simulink model "evitar_choque2023v"  (R2023b)
settings: Solver=VariableStepAuto  StartTime=0.0  StopTime=10.0  RelTol=1e-3
settings Model: Creator=Usuario_UMA  LastModifiedBy=juana

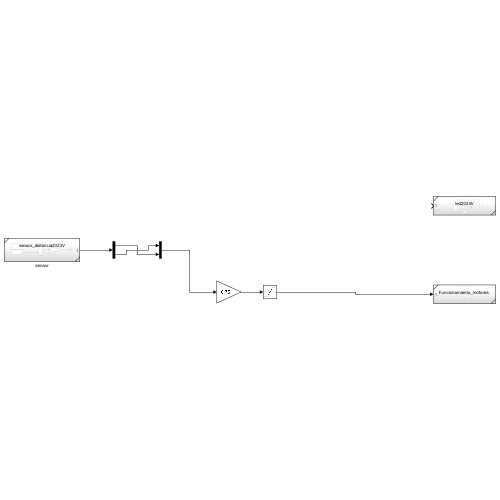
[thumbnail: Simulink's stored preview of the top-level diagram]
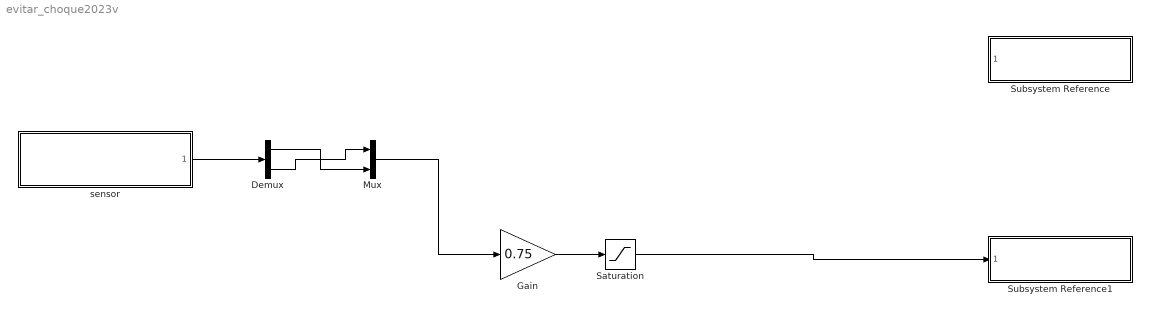
== system evitar_choque2023v ==
  Demux : Demux  Outputs=2
  Gain : Gain  Gain=0.75
  Mux : Mux  Inputs=2
  Saturation : Saturate
  Subsystem Reference : Subsystem  ReferencedSubsystem=led2023V
  Subsystem Reference1 : Subsystem  ReferencedSubsystem=Funcionamiento_motores
  sensor : Subsystem  ReferencedSubsystem=sensor_distancia2023V
  wires:
  sensor/1 -> Demux/1
  Demux/1 -> Mux/2
  Demux/2 -> Mux/1
  Mux/1 -> Gain/1
  Gain/1 -> Saturation/1
  Saturation/1 -> Subsystem Reference1/1
